simulink model "Power_Window_DCMotor_Control_Design"  (R2014a)
settings: Solver=ode15s  StartTime=0.0  StopTime=5  RelTol=1e-3
PreLoadFcn:
  | DC_Motor_R = 0.15;
  | DC_Motor_L = 0.036;
  | DC_Motor_K = 8;
  | DC_Motor_J = 0.085;
  | DC_Motor_B = 5;
  | 
  | PWin_Gain = 1;
  | PWin_Zero = 4;
  | 
libraries: fl_lib x11, nesl_utility x4
Description:
  | Copyright 2014 The MathWorks, Inc.
settings Model: Creator=smiller  LastModifiedBy=smiller
settings DataIOCC: SignalLoggingName=DataLog
settings OptimizationCC: ExpressionDepthLimit=2147483647  InitFltsAndDblsToZero=on
settings DebuggingCC: AlgebraicLoopMsg=none  SaveWithParameterizedLinksMsg=none  UnderspecifiedInitializationDetection=Classic  SolverPrmCheckMsg=none  FcnCallInpInsideContextMsg=UseLocalSettings  UnconnectedInputMsg=none  UnconnectedOutputMsg=none  UnconnectedLineMsg=none  StateNameClashWarn=warning
settings GRTTargetCC: TargetFcnLib=ansi_tfl_tmw.mat  CombineOutputUpdateFcns=off  GRTInterface=on

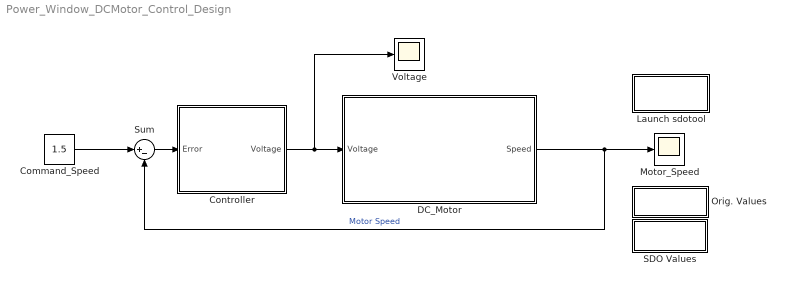
== system Power_Window_DCMotor_Control_Design ==
  Command_Speed : Constant  Value=1.5
  Controller : Subsystem
  DC_Motor : Subsystem
      mask Display:
      | image(imread('Simscape_DC_Motor.jpg'));
      | port_label('Input',1,'Voltage');
      | port_label('Output',1,'Speed');
  Launch sdotool : Subsystem
      settings: OpenFcn=|
      | load([bdroot '_sdosession']);
      | sdotool(SDOSessionData);
      mask Display: disp('Launch\nsdotool')
  Motor_Speed : Scope
      settings: YMin=0  YMax=2  SaveName=PWin_SCD_DATA
  Orig. Values : Subsystem
      settings: OpenFcn=|
      | PWin_Gain = 1;
      | PWin_Zero = 4;
      mask Display: disp('Orig. Values')
  SDO Values : Subsystem
      settings: OpenFcn=|
      | PWin_Gain = 25.0119;
      | PWin_Zero = 0.2911;
      mask Display: disp('SDO Values')
  Sum : Sum  Inputs=|+-
  Voltage : Scope
      settings: YMin=0  SaveName=FEL_Arm_Angle_DATA1
  wires:
  Controller/1(Voltage) -> DC_Motor/1(Voltage), Voltage/1
  DC_Motor/1(Speed) -> Sum/2, Motor_Speed/1  "Motor Speed"
  Command_Speed/1 -> Sum/1
  Sum/1 -> Controller/1(Error)

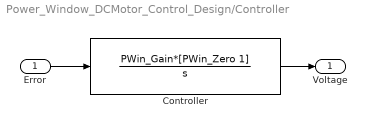
== system Power_Window_DCMotor_Control_Design/Controller ==
  Error : Inport
  Controller : TransferFcn  Numerator=PWin_Gain*[PWin_Zero 1]  Denominator=[1 0]
  Voltage : Outport
  wires:
  Error/1 -> Controller/1
  Controller/1 -> Voltage/1

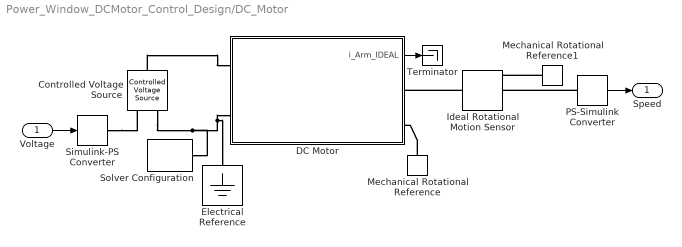
== system Power_Window_DCMotor_Control_Design/DC_Motor ==
  Voltage : Inport
  Controlled Voltage Source : fl_lib/Electrical/Electrical Sources/Controlled Voltage Source
  DC Motor : Subsystem
      mask Display:
      | image(imread('Simscape_DC_Motor.jpg'));
      | port_label('lconn',1,'V+');
      | port_label('lconn',2,'V-');
      | port_label('rconn',1,'Shaft');
      | port_label('rconn',2,'Housing');
      | port_label('Output',1,'i_Arm');
  Electrical Reference : fl_lib/Electrical/Electrical Elements/Electrical Reference
  Ideal Rotational Motion Sensor : fl_lib/Mechanical/Mechanical Sensors/Ideal Rotational Motion Sensor  offset=0 rad
  Mechanical Rotational Reference : fl_lib/Mechanical/Rotational Elements/Mechanical Rotational Reference
  Mechanical Rotational Reference1 : fl_lib/Mechanical/Rotational Elements/Mechanical Rotational Reference
  PS-Simulink Converter : nesl_utility/PS-Simulink Converter  PhysicalDomain=network_engine_domain  SubClassName=ps_output  LeftPortType=input  RightPortType=output  PseudoPeriodic=off  Frequencies=[]  Unit=1  AffineConversion=off
  Simulink-PS Converter : nesl_utility/Simulink-PS Converter  PhysicalDomain=network_engine_domain  SubClassName=ps_input  LeftPortType=input  RightPortType=output  PseudoPeriodic=off  Frequencies=[]  NoiseDistribution=none  NoiseParameters=[]  Unit=1  AffineConversion=off  InputFiltering=off  SimscapeFilterOrder=1  InputFilterTimeConstant=.001  UdotUserProvided=0
  Solver Configuration : nesl_utility/Solver Configuration  PhysicalDomain=network_engine_domain  SubClassName=solver  LeftPortType=input  RightPortType=generic  Accelerate=off  Tones=[]  Harmonics=[]  SimulateNoise=off  Profile=off  UseLocalSampling=off  EnableSwitchedLinearOptims=on  FrequencyDomain=off  UseCCode=off  RelTol=0.001  AbsTol=1e-06  MinStep=1e-09  ToWorkspace=off  DoDC=off  ResidualTolerance=1e-9  UseLocalSolver=off  LocalSolverChoice=NE_BACKWARD_EULER_ADVANCER  LocalSolverSampleTime=.001  DoFixedCost=off  MaxNonlinIter=12  MaxModeIter=2  LinearAlgebra=Sparse  DelaysMemoryBudget=1024  AutomaticFiltering=on  FilteringTimeConstant=0.001
  Terminator : Terminator
  Speed : Outport
  wires:
  DC Motor/1(i_Arm_IDEAL) -> Terminator/1
  PS-Simulink Converter/1 -> Speed/1
  Voltage/1 -> Simulink-PS Converter/1
  connections:
  Controlled Voltage Source/LConn1 -- DC Motor/LConn1
  Simulink-PS Converter/RConn1 -- Controlled Voltage Source/RConn1
  Controlled Voltage Source/RConn2 -- Solver Configuration/RConn1 -- DC Motor/LConn2 -- Electrical Reference/LConn1
  Ideal Rotational Motion Sensor/LConn1 -- DC Motor/RConn1
  Mechanical Rotational Reference/LConn1 -- DC Motor/RConn2
  Mechanical Rotational Reference1/LConn1 -- Ideal Rotational Motion Sensor/RConn1
  PS-Simulink Converter/LConn1 -- Ideal Rotational Motion Sensor/RConn2

== system Power_Window_DCMotor_Control_Design/Launch sdotool ==

== system Power_Window_DCMotor_Control_Design/Orig. Values ==

== system Power_Window_DCMotor_Control_Design/SDO Values ==

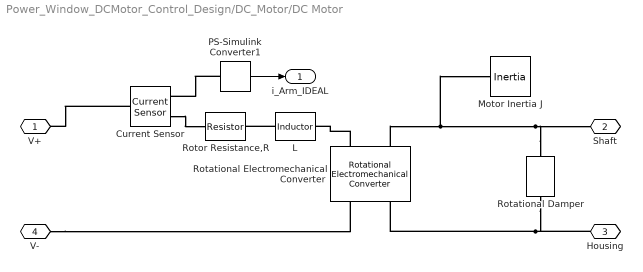
== system Power_Window_DCMotor_Control_Design/DC_Motor/DC Motor ==
  Current Sensor : fl_lib/Electrical/Electrical Sensors/Current Sensor
  L : fl_lib/Electrical/Electrical Elements/Inductor  l=DC_Motor_L H  r=0 Ohm  g=1e-09 1/Ohm  i_specify=off  i_priority=High  i=0 A  v_specify=off  v_priority=High  v=0 V  i_L_specify=on  i_L_priority=High  i_L=0 A
  Motor Inertia J : fl_lib/Mechanical/Rotational Elements/Inertia  inertia=DC_Motor_J kg*m^2  w_specify=on  w_priority=High  w=0 rad/s  t_specify=off  t_priority=High  t=0 N*m
  PS-Simulink Converter1 : nesl_utility/PS-Simulink Converter  PhysicalDomain=network_engine_domain  SubClassName=ps_output  LeftPortType=input  RightPortType=output  PseudoPeriodic=off  Frequencies=[]  Unit=A  AffineConversion=off
  Rotational Electromechanical Converter : fl_lib/Electrical/Electrical Elements/Rotational Electromechanical Converter  K=DC_Motor_K V/(rad/s)  i_specify=off  i_priority=High  i=0 A  v_specify=off  v_priority=High  v=0 V  t_specify=off  t_priority=High  t=0 N*m  w_specify=off  w_priority=High  w=0 rad/s
  Rotational Damper : fl_lib/Mechanical/Rotational Elements/Rotational Damper  D=DC_Motor_B N*m/(rad/s)  w_specify=off  w_priority=High  w=0 rad/s  t_specify=off  t_priority=High  t=0 N*m
  Rotor Resistance,R : fl_lib/Electrical/Electrical Elements/Resistor  Tag=Factory Generic  R=DC_Motor_R Ohm  i_specify=off  i_priority=High  i=0 A  v_specify=off  v_priority=High  v=0 V
  V+ : PMIOPort  Port=1  Side=Left
  Shaft : PMIOPort  Port=2  Side=Right
  Housing : PMIOPort  Port=3  Side=Right
  V- : PMIOPort  Port=4  Side=Left
  i_Arm_IDEAL : Outport
  wires:
  PS-Simulink Converter1/1 -> i_Arm_IDEAL/1
  connections:
  PS-Simulink Converter1/LConn1 -- Current Sensor/RConn1
  Current Sensor/RConn2 -- Rotor Resistance,R/LConn1
  Current Sensor/LConn1 -- V+/RConn1
  Rotational Electromechanical Converter/LConn1 -- L/RConn1
  V-/RConn1 -- Rotational Electromechanical Converter/RConn1
  L/LConn1 -- Rotor Resistance,R/RConn1
  Rotational Damper/LConn1 -- Shaft/RConn1 -- Motor Inertia J/LConn1 -- Rotational Electromechanical Converter/LConn2
  Rotational Damper/RConn1 -- Rotational Electromechanical Converter/RConn2 -- Housing/RConn1
